simulink model "NLGC_1"  (R2017b)
settings: Solver=ode45  StartTime=0.0  StopTime=45  FixedStep=0.05  MaxStep=0.06  RelTol=1e-3  EnableMultiTasking=on
model workspace (MAT data in the model file):
  Sig = Simulink.Signal
  Sig.DataType = 'auto'
  Sig.Dimensions = -1
  Sig.DimensionsMode = 'auto'
  Sig.Complexity = 'auto'
  Sig.SampleTime = -1
  Sig.SamplingMode = 'auto'
undefined symbols (not defined in the file): IC, quadModel
libraries: simulink x4
Description:
  | This is a configurable quadcopter simulation.
  | This Simulink model demonstates position control.
  | 
  | Additional quadcopter modeling and simulation materials available at:
  | github.com/dch33/Quad-Sim
  | 
  | Copyright (C) 2014 D. Hartman, K. Landis, S. Moreno, J. Kim, M. Mehrer
  | 
  | License:
  |     This program is free software: you can redistribute it and/or modify
  |     it under the terms of the GNU LESSER GENERAL PUBLIC LICENSE as published by
  |     the Free Software Foundation, either version 3 of the License, or
  |     (at your option) any later version.
  | 
  |     This program is distributed in the hope that it will be useful,
  |     but WITHOUT ANY WARRANTY; without even the implied warranty of
  |     MERCHANTABILITY or FITNESS FOR A PARTICULAR PURPOSE.  See the
  |     GNU General Public License for more details.
  | 
  |     You should have received a copy of the GNU LESSER GENERAL PUBLIC LICENSE
  |     along with this program.  If not, see <http://www.gnu.org/licenses/>.
settings Model: ModifiedComment=hoang -- Wed Apr 11 06:13:36 2018 -- Version 1.7  Creator=David Hartman  LastModifiedBy=hoang
settings Model: ModifiedHistory=|
  | hoang -- Wed Apr 11 06:13:36 2018 -- Version 1.7
  | 
  | hoang -- Wed Apr 11 04:36:33 2018 -- Version 1.6
  | 
  | davidhartman -- Fri Jun 06 22:59:54 2014 -- Version 1.5
settings DataIOCC: SaveFormat=Array  SignalLogging=off
settings OptimizationCC: DefaultParameterBehavior=Inlined  LifeSpan=inf
settings DebuggingCC: SolverPrmCheckMsg=warning  UniqueDataStoreMsg=warning  StateNameClashWarn=warning  StrictBusMsg=ErrorOnBusTreatedAsVector  SFUnexpectedBacktrackingDiag=warning  SFNoUnconditionalDefaultTransitionDiag=warning  SFExecutionAtInitializationDiag=none
settings HardwareCC: ProdBitPerPointer=32  ProdBitPerSizeT=32  ProdBitPerPtrDiffT=32  ProdLargestAtomicFloat=None  ProdIntDivRoundTo=Undefined  ProdEndianess=Unspecified  ProdWordSize=32  ProdHWDeviceType=32-bit Generic
settings ModelReferenceCC: PropagateSignalLabelsOutOfModel=off
settings CodeAppCC: StateflowObjectComments=on
settings GRTTargetCC: TargetLangStandard=C89/C90 (ANSI)  GeneratePreprocessorConditionals=Disable all
settings ConfigComp: CovMetricSettings=dw  CovHtmlReporting=on  CovSaveCumulativeToWorkspaceVar=on  CovSaveSingleToWorkspaceVar=on  CovExternalEMLEnable=off

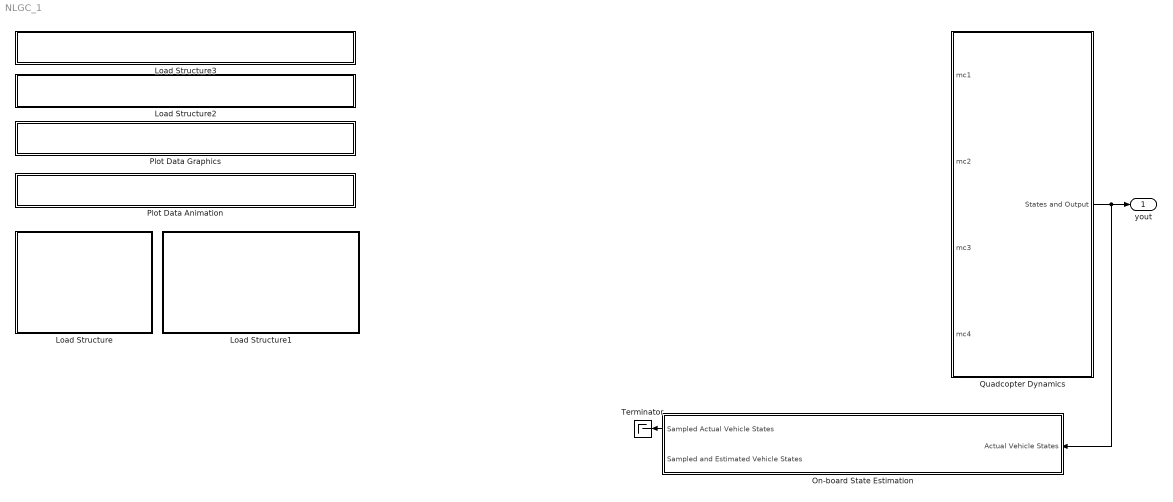
== system NLGC_1 ==
  Load Structure : Subsystem
      settings: OpenFcn=|
      | uiopen('load')
      | if ((exist('IC')==1) && (exist('quadModel')==1) && (exist('path')==1))
      | set_param(bdroot, 'SimulationCommand', 'update')
      | end
      mask Display: fprintf('LOAD:\nTimeseries\nPath\nCommands,\nQuadcopter\nModel, Or\nInitial\nConditions');
  Load Structure1 : Subsystem
      settings: OpenFcn=|
      | if (exist('IC')==1 && exist('quadModel')==1 && exist('yout') && exist('tout'))
      | saveSimResults()
      | else
      | msgbox('No Data To Save!')
      | end
      mask Display: fprintf('SAVE:\nSimulation\nResults');
  Load Structure2 : Subsystem
      settings: OpenFcn=|
      | if exist('GUI_Modeling') == 2,
      | run('GUI_Modeling')
      | 
      | else
      | 
      | msgbox('The desired GUI must be first added to MATLABs path.')
      | 
      | end
      mask Display: fprintf('OPEN GUI: Build New \n Model');
  Load Structure3 : Subsystem
      settings: OpenFcn=|
      | if exist('GUI_IC') == 2,
      | run('GUI_IC')
      | 
      | else
      | 
      | msgbox('The desired GUI must be first added to MATLABs path.')
      | 
      | end
      mask Display: fprintf('OPEN GUI: Create Initial \n Conditions');
  On-board State Estimation : Subsystem  mask{ControllerSampleTime=1/350, Gyro_Alpha=0.50, Accel_Alpha=0.06, EAComp=0.92}
      mask prompts: ControllerSampleTime "State sensor sampling time (s):"; Gyro_Alpha "Gyro Alpha Value:"; Accel_Alpha "Accelerometer Alpha Value:"; EAComp "Complimentary Filter Alpha (must be between 0 and 1):"
      mask Help:
      | Sampling Time: A typical value might be 0.02 to 0.002 seconds (50 Hz to 400 Hz)
      | depending on the control system and sensors used. For best simulink performance,
      | it may be necessarry to round the value a bit to achieve an integer multiple
      | relationship between motor command sampling time and state estimation sampling time.
      | See simulink documentation for more details.
      mask TypeOptions ControllerSampleTime: Rate Transition/OutPortSampleTime
      mask TypeOptions Gyro_Alpha: filterRawData()/Gyro_Alpha
      mask TypeOptions Accel_Alpha: filterRawData()/Accel_Alpha
      mask TypeOptions EAComp: State Estimation and Complimentary Mixing/EAComp
      mask Display:
      | fprintf(['Sampling Time: ' num2str(ControllerSampleTime) ' (s)']);
      | fprintf(['\n \n' num2str(1/ControllerSampleTime) ' Hz']);
  Plot Data Animation : Subsystem
      settings: OpenFcn=|
      | if exist('QuadAnim4') == 2,
      |     if exist('yout')
      | 	run('QuadAnim4');
      |     else
      |     msgbox('Simulation must be run before data can be plotted.');
      |     end
      | else                                                                          msgbox('The desired GUI must be first added to MATLABs path.')
      | end
      mask Display: fprintf('OPEN GUI: Flight Animation')
  Plot Data Graphics : Subsystem
      settings: OpenFcn=|
      | if exist('yout')
      | yout = evalin('base', 'yout');
      | tout = evalin('base', 'tout');
      | quadPlots(yout, tout)
      | else
      | msgbox('Simulation must be run before data can be plotted.')
      | end
      mask Display: fprintf('OPEN PLOT: State Data')
  Quadcopter Dynamics : Subsystem
  Terminator : Terminator
  yout : Outport
  wires:
  Quadcopter Dynamics/1(States and Output) -> yout/1, On-board State Estimation/1(Actual Vehicle States)
  On-board State Estimation/1(Sampled Actual Vehicle States) -> Terminator/1

== system NLGC_1/Load Structure ==

== system NLGC_1/Load Structure1 ==

== system NLGC_1/Load Structure2 ==

== system NLGC_1/Load Structure3 ==

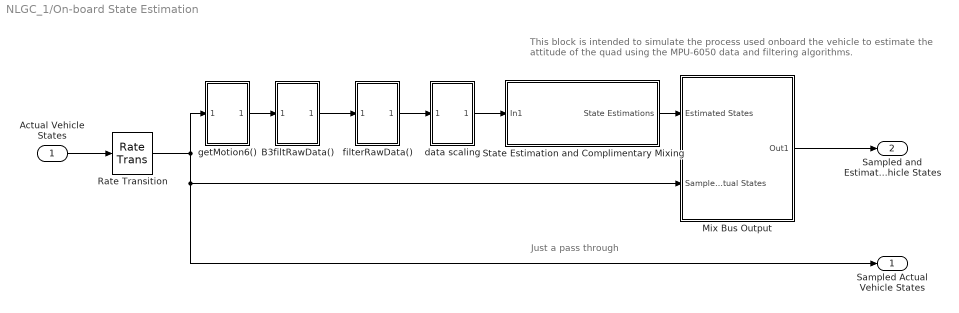
== system NLGC_1/On-board State Estimation ==
  note: This block is intended to simulate the process used onboard the vehicle
      | to estimate the attitude of the quad using the MPU-6050 data and filtering algorithms.
  note: Just a pass through
  Actual Vehicle States : Inport
  B3filtRawData() : Subsystem  mask{inputGain=1/3.102185882e+03, x1x2Gain=3, y2Gain=2.7130114176, y1Gain=-2.4657422174, y0Gain=0.7501519731}
      mask prompts: inputGain "Input Gain:"; x1x2Gain "x1x2 Gain:"; y2Gain "y2 Gain:"; y1Gain "y1 Gain:"; y0Gain "y0 Gain:"
      mask TypeOptions inputGain: InputGain/Gain
      mask TypeOptions x1x2Gain: x1x2Gain/Gain
      mask TypeOptions y2Gain: y2Gain/Gain
      mask TypeOptions y1Gain: y1Gain/Gain
      mask TypeOptions y0Gain: y0Gain/Gain
  Mix Bus Output : Subsystem
  Rate Transition : RateTransition  Deterministic=off  OutPortSampleTime=ControllerSampleTime
  State Estimation and Complimentary Mixing : Subsystem  mask{EAComp=EAComp}
      mask prompts: EAComp "Complimentary Filter Alpha:"
      mask TypeOptions EAComp: Complimentary Filter/EAComp
  data scaling : Subsystem
  filterRawData() : Subsystem  mask{Gyro_Alpha=Gyro_Alpha, Accel_Alpha=Accel_Alpha}
      mask prompts: Gyro_Alpha "Gyro Alpha Value:"; Accel_Alpha "Accelerometer Alpha Value:"
      mask TypeOptions Gyro_Alpha: Gyro alpha/Gain
      mask TypeOptions Accel_Alpha: Accel alpha/Gain
  getMotion6() : Subsystem
  Sampled Actual Vehicle States : Outport
  Sampled and Estimated Vehicle States : Outport  Port=2
  wires:
  Actual Vehicle States/1 -> Rate Transition/1
  Rate Transition/1 -> getMotion6()/1(In1), Sampled Actual Vehicle States/1, Mix Bus Output/2(Sampled Actual States)
  getMotion6()/1(Out1) -> B3filtRawData()/1(In1)
  data scaling/1(Out1) -> State Estimation and Complimentary Mixing/1(In1)
  State Estimation and Complimentary Mixing/1(State Estimations) -> Mix Bus Output/1(Estimated States)
  Mix Bus Output/1(Out1) -> Sampled and Estimated Vehicle States/1
  B3filtRawData()/1(Out1) -> filterRawData()/1(In1)
  filterRawData()/1(Out1) -> data scaling/1(In1)

== system NLGC_1/Plot Data Animation ==

== system NLGC_1/Plot Data Graphics ==

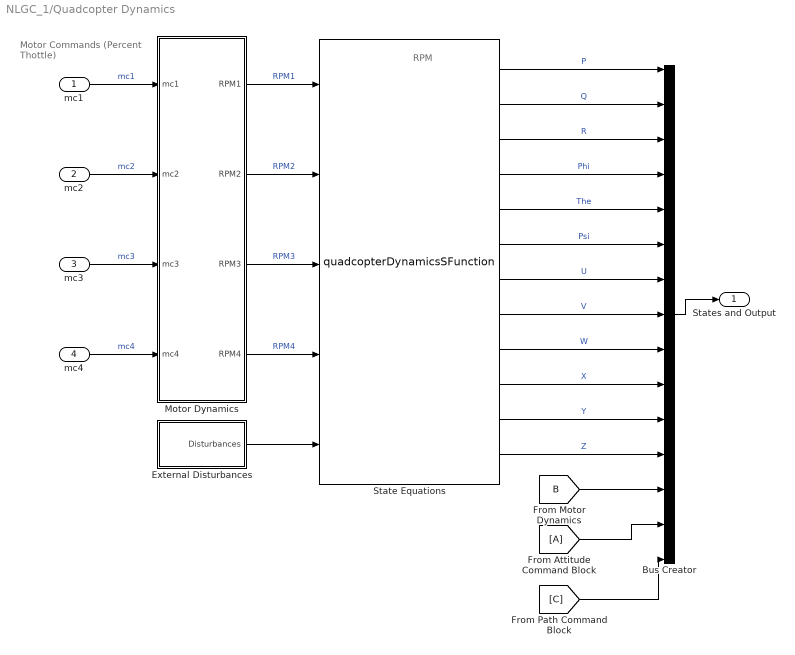
== system NLGC_1/Quadcopter Dynamics ==
  note: RPM
  note: Motor Commands
      | (Percent Thottle)
  mc1 : Inport
  mc2 : Inport  Port=2
  mc3 : Inport  Port=3
  mc4 : Inport  Port=4
  Bus Creator : BusCreator  Inputs='P','Q','R','Phi','The','Psi','U','V','W','X','Y','Z','mc and RPM','Attitude_Cmd','XY_Cmd'
  External Disturbances : Subsystem
  Motor Dynamics : Subsystem
  State Equations : M-S-Function  FunctionName=quadcopterDynamicsSFunction  Parameters=quadModel, IC
      mask Display:
      | port_label('input', 1, 'RPM1')
      | port_label('input', 2, 'RPM2')
      | port_label('input', 3, 'RPM3')
      | port_label('input', 4, 'RPM4')
      | port_label('input', 5, 'Disturbances')
      | port_label('output', 1, 'P')
      | port_label('output', 2, 'Q')
      | port_label('output', 3, 'R')
      | port_label('output', 4, 'Phi')
      | port_label('output', 5, 'The')
      | port_label('output', 6, 'Psi')
      | port_label('output', 7, 'U')
      | port_label('output', 8, 'V')
      | port_label('output', 9, 'W')
      | port_label('output', 10, 'X')
      | port_label('output', 11, 'Y')
      | port_label('output', 12, 'Z')
  States and Output : Outport
  wires:
  State Equations/1 -> Bus Creator/1  "P"
  State Equations/2 -> Bus Creator/2  "Q"
  State Equations/3 -> Bus Creator/3  "R"
  State Equations/4 -> Bus Creator/4  "Phi"
  State Equations/5 -> Bus Creator/5  "The"
  State Equations/6 -> Bus Creator/6  "Psi"
  State Equations/7 -> Bus Creator/7  "U"
  State Equations/8 -> Bus Creator/8  "V"
  State Equations/9 -> Bus Creator/9  "W"
  State Equations/10 -> Bus Creator/10  "X"
  State Equations/11 -> Bus Creator/11  "Y"
  State Equations/12 -> Bus Creator/12  "Z"
  Bus Creator/1 -> States and Output/1
  Motor Dynamics/1(RPM1) -> State Equations/1  "RPM1"
  Motor Dynamics/2(RPM2) -> State Equations/2  "RPM2"
  Motor Dynamics/3(RPM3) -> State Equations/3  "RPM3"
  Motor Dynamics/4(RPM4) -> State Equations/4  "RPM4"
  mc1/1 -> Motor Dynamics/1(mc1)  "mc1"
  mc4/1 -> Motor Dynamics/4(mc4)  "mc4"
  mc3/1 -> Motor Dynamics/3(mc3)  "mc3"
  mc2/1 -> Motor Dynamics/2(mc2)  "mc2"
  External Disturbances/1("Disturbances ") -> State Equations/5
  [A] -> Bus Creator/14
  [B] -> Bus Creator/13
  [C] -> Bus Creator/15

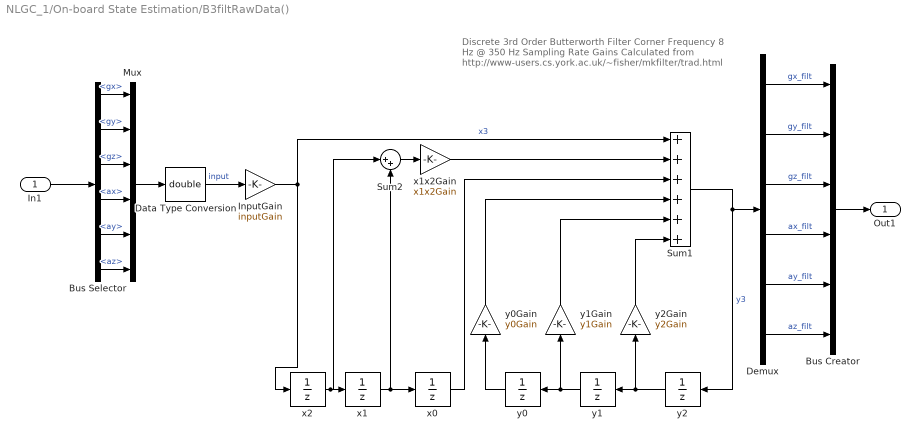
== system NLGC_1/On-board State Estimation/B3filtRawData() ==
  note: Discrete
      | 3rd Order Butterworth Filter
      | Corner Frequency 8 Hz @ 350 Hz Sampling Rate
      | Gains Calculated from
      | http://www-users.cs.york.ac.uk/~fisher/mkfilter/trad.html
  In1 : Inport
  Bus Creator : BusCreator  Inputs=6
  Bus Selector : BusSelector  OutputSignals=gx,gy,gz,ax,ay,az
  Data Type Conversion : DataTypeConversion  OutDataTypeStr=double  RndMeth=Nearest
  Demux : Demux  Outputs=6
  InputGain : Gain  Gain=inputGain
  Mux : Mux  Inputs=6
  Sum1 : Sum  Inputs=++++++
  Sum2 : Sum  Inputs=|++
  x0 : UnitDelay  SampleTime=-1
  x1 : UnitDelay  SampleTime=-1
  x1x2Gain : Gain  Gain=x1x2Gain
  x2 : UnitDelay  SampleTime=-1
  y0 : UnitDelay  SampleTime=-1
  y0Gain : Gain  Gain=y0Gain
  y1 : UnitDelay  SampleTime=-1
  y1Gain : Gain  Gain=y1Gain
  y2 : UnitDelay  SampleTime=-1
  y2Gain : Gain  Gain=y2Gain
  Out1 : Outport
  wires:
  Sum1/1 -> Demux/1, y2/1  "y3"
  In1/1 -> Bus Selector/1
  Bus Selector/1 -> Mux/1  "<gx>"
  Bus Selector/2 -> Mux/2  "<gy>"
  Bus Selector/3 -> Mux/3  "<gz>"
  Mux/1 -> Data Type Conversion/1
  Demux/1 -> Bus Creator/1  "gx_filt"
  Demux/2 -> Bus Creator/2  "gy_filt"
  Demux/3 -> Bus Creator/3  "gz_filt"
  Bus Creator/1 -> Out1/1
  Data Type Conversion/1 -> InputGain/1  "input"
  Bus Selector/4 -> Mux/4  "<ax>"
  Bus Selector/5 -> Mux/5  "<ay>"
  Bus Selector/6 -> Mux/6  "<az>"
  Demux/4 -> Bus Creator/4  "ax_filt"
  Demux/5 -> Bus Creator/5  "ay_filt"
  Demux/6 -> Bus Creator/6  "az_filt"
  y2/1 -> y2Gain/1, y1/1
  y1/1 -> y1Gain/1, y0/1
  InputGain/1 -> x2/1, Sum1/1  "x3"
  x2/1 -> Sum2/1, x1/1
  x1/1 -> Sum2/2, x0/1
  Sum2/1 -> x1x2Gain/1
  x1x2Gain/1 -> Sum1/2
  y0Gain/1 -> Sum1/4
  y0/1 -> y0Gain/1
  y1Gain/1 -> Sum1/5
  y2Gain/1 -> Sum1/6
  x0/1 -> Sum1/3

== system NLGC_1/On-board State Estimation/Mix Bus Output ==
  note: These states are sampled actual values
      | not used by the stability controller
  note: These are the estimated states
  Estimated States : Inport
  Sampled Actual States : Inport  Port=2
  Bus Creator : BusCreator  Inputs=12
  Bus Selector1 : BusSelector  OutputSignals=U,V,W,X,Y,Z
  Bus Selector2 : BusSelector  OutputSignals=P,Q,R,Phi,The,Psi
  Debug Scopes For Comparing Actual Versus Estimated Outputs This illustrates some of the effects from filtering : Subsystem
  Out1 : Outport
  wires:
  Bus Selector2/2 -> Bus Creator/2  "<Q>"
  Bus Selector2/3 -> Bus Creator/3  "<R>"
  Bus Selector2/1 -> Bus Creator/1  "<P>"
  Bus Selector2/5 -> Bus Creator/5  "<The>"
  Bus Selector1/5 -> Bus Creator/11  "<Y>"
  Bus Selector1/4 -> Bus Creator/10  "<X>"
  Bus Selector1/1 -> Bus Creator/7  "<U>"
  Estimated States/1 -> Debug Scopes For Comparing Actual Versus Estimated Outputs This illustrates some of the effects from filtering/1(Estimated), Bus Selector2/1
  Bus Selector2/4 -> Bus Creator/4  "<Phi>"
  Bus Selector1/2 -> Bus Creator/8  "<V>"
  Bus Selector1/6 -> Bus Creator/12  "<Z>"
  Bus Creator/1 -> Out1/1
  Sampled Actual States/1 -> Debug Scopes For Comparing Actual Versus Estimated Outputs This illustrates some of the effects from filtering/2(Actual), Bus Selector1/1
  Bus Selector1/3 -> Bus Creator/9  "<W>"
  Bus Selector2/6 -> Bus Creator/6  "<Psi>"

== system NLGC_1/On-board State Estimation/State Estimation and Complimentary Mixing ==
  note: The specific state estimation procedure employed in these bocks is
      | to be considered experimental (like everything else in this simulation).
      | While functional within the context of our application, this is not to be taken
      | as a "correct" method for state estimation or gyro/accelerometer data combination.
  note: Note:
      | x_gyro is taken as P,
      | y_gyro as Q,
      | z_gyro ad R.
  In1 : Inport
  Bus Creator : BusCreator  Inputs=6
  Bus Selector : BusSelector  OutputSignals=P,Q,R,x_acc,y_acc,z_acc
  Complimentary Filter : Subsystem  mask{EAComp=EAComp}
      mask prompts: EAComp "Complimentary Filter Alpha:"
      mask TypeOptions EAComp: EAComp1/Gain
  Subsystem : Subsystem
  Subsystem1 : Subsystem
  State Estimations : Outport
  wires:
  In1/1 -> Bus Selector/1
  Bus Selector/1 -> Bus Creator/4, Subsystem/3(P)  "<P>"
  Bus Selector/3 -> Bus Creator/6, Subsystem/5(R)  "<R>"
  Bus Selector/2 -> Bus Creator/5, Subsystem/4(Q)  "<Q>"
  Subsystem/2(thetaDot_gyro) -> Complimentary Filter/2(theDot_gyro)  "thateDot_gyro"
  Subsystem/3(psiDot_gyro) -> Complimentary Filter/3(psiDot_gyro)  "psiDot_gyro"
  Subsystem/1(phiDot_gyro) -> Complimentary Filter/1(phiDot_gyro)  "phiDot_gyro"
  Complimentary Filter/1(phi_est) -> Bus Creator/1, Subsystem/1(Phi)  "Phi"
  Complimentary Filter/2(theta_est) -> Bus Creator/2, Subsystem/2(Theta)  "The"
  Complimentary Filter/3(psi_est) -> Bus Creator/3  "Psi"
  Subsystem1/2(phi_acc) -> Complimentary Filter/5(phiDot_acc)  "phi_acc"
  Subsystem1/1(theta_acc) -> Complimentary Filter/4(the_acc)  "theta_acc"
  Bus Selector/4 -> Subsystem1/1(x_acc)  "<x_acc>"
  Bus Selector/5 -> Subsystem1/2(y_acc)  "<y_acc>"
  Bus Selector/6 -> Subsystem1/3(z_acc)  "<z_acc>"
  Bus Creator/1 -> State Estimations/1

== system NLGC_1/On-board State Estimation/data scaling ==
  note: For simulation, no
      | offset value is calculated.
  In1 : Inport
  Bus Creator : BusCreator  Inputs=6
  Bus Selector : BusSelector  OutputSignals=gx_filt,gy_filt,gz_filt,ax_filt,ay_filt,az_filt
  Demux : Demux  Outputs=3
  Demux1 : Demux  Outputs=3
  Gain : Gain  Gain=pi/(180*131)
  Gain1 : Gain  Gain=9.81*16384
  Mux1 : Mux  Inputs=3
  Mux2 : Mux  Inputs=3
  Out1 : Outport
  wires:
  In1/1 -> Bus Selector/1
  Bus Selector/1 -> Mux1/1  "<gx_filt>"
  Bus Selector/2 -> Mux1/2  "<gy_filt>"
  Bus Selector/3 -> Mux1/3  "<gz_filt>"
  Bus Selector/4 -> Mux2/1  "<ax_filt>"
  Bus Selector/5 -> Mux2/2  "<ay_filt>"
  Bus Selector/6 -> Mux2/3  "<az_filt>"
  Mux2/1 -> Gain1/1
  Mux1/1 -> Gain/1
  Gain1/1 -> Demux1/1
  Gain/1 -> Demux/1
  Demux/1 -> Bus Creator/1  "P"
  Demux/2 -> Bus Creator/2  "Q"
  Demux/3 -> Bus Creator/3  "R"
  Demux1/1 -> Bus Creator/4  "x_acc"
  Demux1/2 -> Bus Creator/5  "y_acc"
  Demux1/3 -> Bus Creator/6  "z_acc"
  Bus Creator/1 -> Out1/1

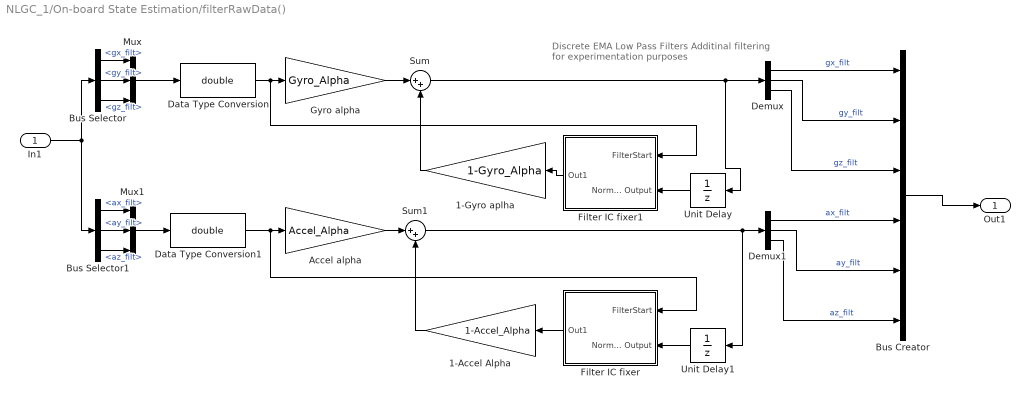
== system NLGC_1/On-board State Estimation/filterRawData() ==
  note: Discrete EMA
      | Low Pass Filters
      | Additinal filtering for experimentation purposes
  In1 : Inport
  1-Accel Alpha : Gain  Gain=1-Accel_Alpha
  1-Gyro aplha : Gain  Gain=1-Gyro_Alpha
  Accel alpha : Gain  Gain=Accel_Alpha
  Bus Creator : BusCreator  Inputs=6
  Bus Selector : BusSelector  OutputSignals=gx_filt,gy_filt,gz_filt
  Bus Selector1 : BusSelector  OutputSignals=ax_filt,ay_filt,az_filt
  Data Type Conversion : DataTypeConversion  OutDataTypeStr=double  RndMeth=Nearest
  Data Type Conversion1 : DataTypeConversion  OutDataTypeStr=double  RndMeth=Nearest
  Demux : Demux  Outputs=3
  Demux1 : Demux  Outputs=3
  Filter IC fixer : Subsystem
  Filter IC fixer1 : Subsystem
  Gyro alpha : Gain  Gain=Gyro_Alpha
  Mux : Mux  Inputs=3
  Mux1 : Mux  Inputs=3
  Sum : Sum  Inputs=|++
  Sum1 : Sum  Inputs=|++
  Unit Delay : UnitDelay  SampleTime=-1
  Unit Delay1 : UnitDelay  SampleTime=-1
  Out1 : Outport
  wires:
  Gyro alpha/1 -> Sum/1
  Sum/1 -> Demux/1, Unit Delay/1
  In1/1 -> Bus Selector1/1, Bus Selector/1
  Accel alpha/1 -> Sum1/1
  1-Gyro aplha/1 -> Sum/2
  1-Accel Alpha/1 -> Sum1/2
  Unit Delay1/1 -> Filter IC fixer/2(Normal Output)
  Filter IC fixer/1(Out1) -> 1-Accel Alpha/1
  Unit Delay/1 -> Filter IC fixer1/2(Normal Output)
  Filter IC fixer1/1(Out1) -> 1-Gyro aplha/1
  Bus Selector/1 -> Mux/1  "<gx_filt>"
  Bus Selector/2 -> Mux/2  "<gy_filt>"
  Bus Selector/3 -> Mux/3  "<gz_filt>"
  Mux/1 -> Data Type Conversion/1
  Demux/1 -> Bus Creator/1  "gx_filt"
  Demux/2 -> Bus Creator/2  "gy_filt"
  Demux/3 -> Bus Creator/3  "gz_filt"
  Bus Creator/1 -> Out1/1
  Mux1/1 -> Data Type Conversion1/1
  Bus Selector1/1 -> Mux1/1  "<ax_filt>"
  Bus Selector1/2 -> Mux1/2  "<ay_filt>"
  Bus Selector1/3 -> Mux1/3  "<az_filt>"
  Sum1/1 -> Unit Delay1/1, Demux1/1
  Demux1/1 -> Bus Creator/4  "ax_filt"
  Demux1/2 -> Bus Creator/5  "ay_filt"
  Demux1/3 -> Bus Creator/6  "az_filt"
  Data Type Conversion/1 -> Filter IC fixer1/1(FilterStart), Gyro alpha/1
  Data Type Conversion1/1 -> Filter IC fixer/1(FilterStart), Accel alpha/1

== system NLGC_1/On-board State Estimation/getMotion6() ==
  note: Simulate getMotion()
  note: Get std measurement from sensor
      | connect to front mask
  In1 : Inport
  Accelerometer : Subsystem
  Bus Creator : BusCreator  Inputs=6
  Bus Selector : BusSelector  OutputSignals=P,Q,R,Phi,The
  Gyro signals : Subsystem
  Out1 : Outport
  wires:
  Bus Selector/2 -> Gyro signals/2(Q)  "<Q>"
  Bus Selector/1 -> Gyro signals/1(P)  "<P>"
  Gyro signals/2(gy) -> Bus Creator/2  "gy"
  Accelerometer/1(ax) -> Bus Creator/4  "ax"
  Bus Selector/5 -> Accelerometer/2(Theta)  "<The>"
  Bus Selector/4 -> Accelerometer/1(Phi)  "<Phi>"
  Bus Selector/3 -> Gyro signals/3(R)  "<R>"
  Gyro signals/1(gx) -> Bus Creator/1  "gx"
  In1/1 -> Bus Selector/1
  Gyro signals/3(gz) -> Bus Creator/3  "gz"
  Accelerometer/2(ay) -> Bus Creator/5  "ay"
  Accelerometer/3(az) -> Bus Creator/6  "az"
  Bus Creator/1 -> Out1/1

== system NLGC_1/Quadcopter Dynamics/External Disturbances ==
  note: Note: Torques are in units of N*m, Forces in N
      | Torques are applied to the BODY coordinate system.
      | Forces are applied from the WORLD coordinate system!
      | This can be changed by adjusting the equations within the S-function.
  Bus Creator : BusCreator  Inputs=6
  Bus to Vector : BusToVector
  Constant{2..6} (5 alike) : Constant  Value=0
  Step : Step  After=0  SampleTime=0
  "Disturbances " : Outport
  wires:
  Bus to Vector/1 -> "Disturbances "/1
  Bus Creator/1 -> Bus to Vector/1
  Constant6/1 -> Bus Creator/1  "Tau_bx-axis"
  Step/1 -> Bus Creator/2  "Tau_by-axis"
  Constant2/1 -> Bus Creator/3  "Tau_bz-axis"
  Constant3/1 -> Bus Creator/4  "Force_x-axis"
  Constant4/1 -> Bus Creator/5  "Force_y-axis"
  Constant5/1 -> Bus Creator/6  "Force_z-axis"

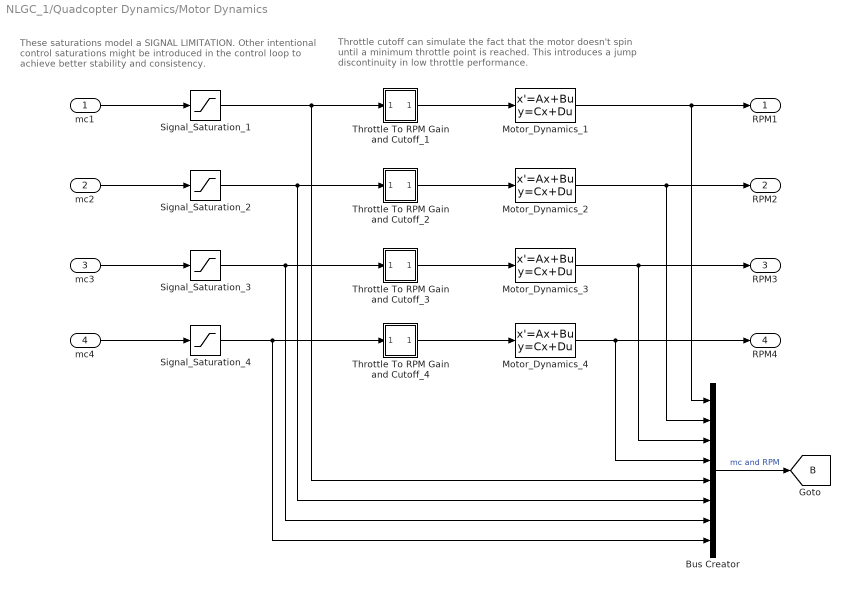
== system NLGC_1/Quadcopter Dynamics/Motor Dynamics ==
  note: Throttle cutoff can simulate the fact that the motor doesn't
      | spin until a minimum throttle point is reached. This introduces
      | a jump discontinuity in low throttle performance.
  note: These saturations model a SIGNAL LIMITATION.
      | Other intentional control saturations might be introduced in the
      | control loop to achieve better stability and consistency.
  mc1 : Inport
  mc2 : Inport  Port=2
  mc3 : Inport  Port=3
  mc4 : Inport  Port=4
  Bus Creator : BusCreator  Inputs=8
  Motor_Dynamics_1 : StateSpace  A=-1/quadModel.T  C=1/quadModel.T  D=0  InitialCondition=IC.w1*quadModel.T
  Motor_Dynamics_2 : StateSpace  A=-1/quadModel.T  C=1/quadModel.T  D=0  InitialCondition=IC.w2*quadModel.T
  Motor_Dynamics_3 : StateSpace  A=-1/quadModel.T  C=1/quadModel.T  D=0  InitialCondition=IC.w3*quadModel.T
  Motor_Dynamics_4 : StateSpace  A=-1/quadModel.T  C=1/quadModel.T  D=0  InitialCondition=IC.w4*quadModel.T
  Signal_Saturation_{1..4} (4 alike) : Saturate  UpperLimit=100  LowerLimit=0
  Throttle To RPM Gain and Cutoff_1 : Subsystem
  Throttle To RPM Gain and Cutoff_2 : Subsystem
  Throttle To RPM Gain and Cutoff_3 : Subsystem
  Throttle To RPM Gain and Cutoff_4 : Subsystem
  RPM1 : Outport
  RPM2 : Outport  Port=2
  RPM3 : Outport  Port=3
  RPM4 : Outport  Port=4
  tag scope: B=global
  wires:
  mc1/1 -> Signal_Saturation_1/1
  mc4/1 -> Signal_Saturation_4/1
  mc2/1 -> Signal_Saturation_2/1
  mc3/1 -> Signal_Saturation_3/1
  Signal_Saturation_1/1 -> Bus Creator/5, Throttle To RPM Gain and Cutoff_1/1(In5)
  Signal_Saturation_2/1 -> Bus Creator/6, Throttle To RPM Gain and Cutoff_2/1(In5)
  Signal_Saturation_3/1 -> Bus Creator/7, Throttle To RPM Gain and Cutoff_3/1(In5)
  Signal_Saturation_4/1 -> Bus Creator/8, Throttle To RPM Gain and Cutoff_4/1(In5)
  Throttle To RPM Gain and Cutoff_1/1(Out5) -> Motor_Dynamics_1/1
  Throttle To RPM Gain and Cutoff_2/1(Out5) -> Motor_Dynamics_2/1
  Throttle To RPM Gain and Cutoff_3/1(Out5) -> Motor_Dynamics_3/1
  Throttle To RPM Gain and Cutoff_4/1(Out5) -> Motor_Dynamics_4/1
  Motor_Dynamics_1/1 -> Bus Creator/1, RPM1/1
  Motor_Dynamics_2/1 -> Bus Creator/2, RPM2/1
  Motor_Dynamics_3/1 -> Bus Creator/3, RPM3/1
  Motor_Dynamics_4/1 -> Bus Creator/4, RPM4/1
  Bus Creator/1 -> [B]  "mc and RPM"

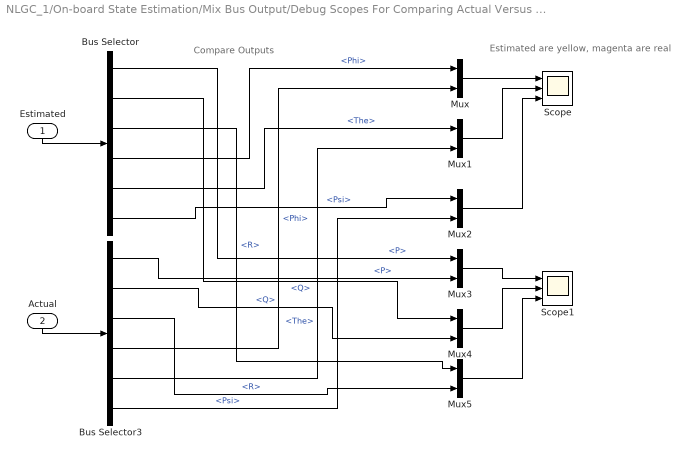
== system NLGC_1/On-board State Estimation/Mix Bus Output/Debug Scopes For Comparing Actual Versus Estimated Outputs This illustrates some of the effects from filtering ==
  note: Estimated are yellow, magenta are real
  note: Compare Outputs
  Estimated : Inport
  Actual : Inport  Port=2
  Bus Selector : BusSelector  OutputSignals=P,Q,R,Phi,The,Psi
  Bus Selector3 : BusSelector  OutputSignals=P,Q,R,Phi,The,Psi
  Mux{,1..5} (6 alike) : Mux  Inputs=2
  Scope : Scope  NumInputPorts=3
  Scope1 : Scope  NumInputPorts=3
  wires:
  Actual/1 -> Bus Selector3/1
  Mux5/1 -> Scope1/3
  Estimated/1 -> Bus Selector/1
  Bus Selector3/2 -> Mux4/2  "<Q>"
  Mux3/1 -> Scope1/1
  Mux4/1 -> Scope1/2
  Bus Selector/1 -> Mux3/1  "<P>"
  Bus Selector3/1 -> Mux3/2  "<P>"
  Bus Selector3/5 -> Mux1/2  "<The>"
  Bus Selector/3 -> Mux5/1  "<R>"
  Bus Selector/6 -> Mux2/1  "<Psi>"
  Bus Selector/2 -> Mux4/1  "<Q>"
  Mux2/1 -> Scope/3
  Bus Selector/5 -> Mux1/1  "<The>"
  Bus Selector/4 -> Mux/1  "<Phi>"
  Bus Selector3/3 -> Mux5/2  "<R>"
  Bus Selector3/6 -> Mux2/2  "<Psi>"
  Mux/1 -> Scope/1
  Mux1/1 -> Scope/2
  Bus Selector3/4 -> Mux/2  "<Phi>"

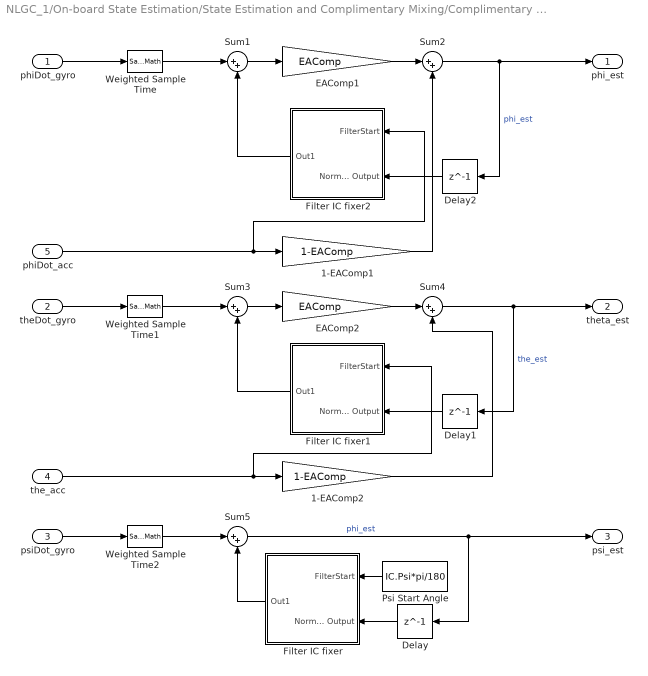
== system NLGC_1/On-board State Estimation/State Estimation and Complimentary Mixing/Complimentary Filter ==
  phiDot_gyro : Inport
  theDot_gyro : Inport  Port=2
  psiDot_gyro : Inport  Port=3
  the_acc : Inport  Port=4
  phiDot_acc : Inport  Port=5
  1-EAComp1 : Gain  Gain=1-EAComp
  1-EAComp2 : Gain  Gain=1-EAComp
  Delay : Delay  DelayLength=1  InitialCondition=0
  Delay1 : Delay  DelayLength=1  InitialCondition=0
  Delay2 : Delay  DelayLength=1  InitialCondition=0
  EAComp1 : Gain  Gain=EAComp
  EAComp2 : Gain  Gain=EAComp
  Filter IC fixer : Subsystem
  Filter IC fixer1 : Subsystem
  Filter IC fixer2 : Subsystem
  Psi Start Angle : Constant  Value=IC.Psi*pi/180
  Sum{1..5} (5 alike) : Sum  Inputs=|++
  Weighted Sample Time : SampleTimeMath  TsampMathOp=*
  Weighted Sample Time1 : SampleTimeMath  TsampMathOp=*
  Weighted Sample Time2 : SampleTimeMath  TsampMathOp=*
  phi_est : Outport
  theta_est : Outport  Port=2
  psi_est : Outport  Port=3
  wires:
  Weighted Sample Time/1 -> Sum1/1
  Sum1/1 -> EAComp1/1
  Sum2/1 -> Delay2/1, phi_est/1  "phi_est"
  1-EAComp1/1 -> Sum2/2
  phiDot_gyro/1 -> Weighted Sample Time/1
  phiDot_acc/1 -> Filter IC fixer2/1(FilterStart), 1-EAComp1/1
  EAComp1/1 -> Sum2/1
  Weighted Sample Time1/1 -> Sum3/1
  Sum3/1 -> EAComp2/1
  Sum4/1 -> Delay1/1, theta_est/1  "the_est"
  1-EAComp2/1 -> Sum4/2
  theDot_gyro/1 -> Weighted Sample Time1/1
  the_acc/1 -> 1-EAComp2/1, Filter IC fixer1/1(FilterStart)
  EAComp2/1 -> Sum4/1
  psiDot_gyro/1 -> Weighted Sample Time2/1
  Weighted Sample Time2/1 -> Sum5/1
  Sum5/1 -> Delay/1, psi_est/1  "phi_est"
  Delay/1 -> Filter IC fixer/2(Normal Output)
  Filter IC fixer/1(Out1) -> Sum5/2
  Psi Start Angle/1 -> Filter IC fixer/1(FilterStart)
  Filter IC fixer1/1(Out1) -> Sum3/2
  Filter IC fixer2/1(Out1) -> Sum1/2
  Delay1/1 -> Filter IC fixer1/2(Normal Output)
  Delay2/1 -> Filter IC fixer2/2(Normal Output)

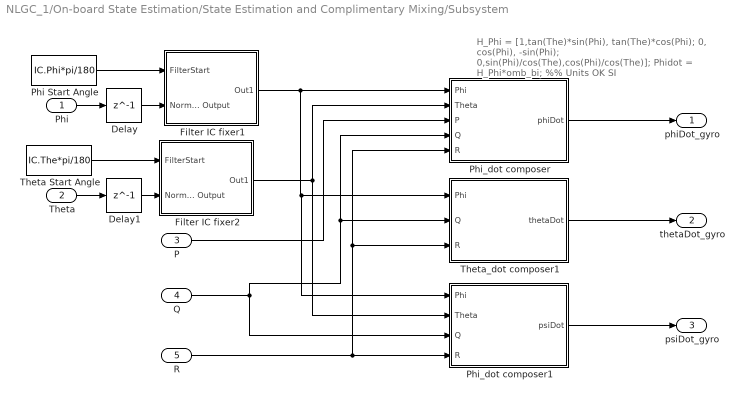
== system NLGC_1/On-board State Estimation/State Estimation and Complimentary Mixing/Subsystem ==
  note: H_Phi = [1,tan(The)*sin(Phi), tan(The)*cos(Phi);
      |          0,         cos(Phi),         -sin(Phi);
      |          0,sin(Phi)/cos(The),cos(Phi)/cos(The)];
      | Phidot = H_Phi*omb_bi; %% Units OK SI
  Phi : Inport
  Theta : Inport  Port=2
  P : Inport  Port=3
  Q : Inport  Port=4
  R : Inport  Port=5
  Delay : Delay  DelayLength=1  InitialCondition=0
  Delay1 : Delay  DelayLength=1  InitialCondition=0
  Filter IC fixer1 : Subsystem
  Filter IC fixer2 : Subsystem
  Phi Start Angle : Constant  Value=IC.Phi*pi/180
  Phi_dot composer : Subsystem
  Phi_dot composer1 : Subsystem
  Theta Start Angle : Constant  Value=IC.The*pi/180
  Theta_dot composer1 : Subsystem
  phiDot_gyro : Outport
  thetaDot_gyro : Outport  Port=2
  psiDot_gyro : Outport  Port=3
  wires:
  P/1 -> Phi_dot composer/3(P)
  Q/1 -> Phi_dot composer1/3(Q), Theta_dot composer1/2(Q), Phi_dot composer/4(Q)
  Phi_dot composer/1(phiDot) -> phiDot_gyro/1
  Theta_dot composer1/1(thetaDot) -> thetaDot_gyro/1
  R/1 -> Theta_dot composer1/3(R), Phi_dot composer/5(R), Phi_dot composer1/4(R)
  Phi_dot composer1/1(psiDot) -> psiDot_gyro/1
  Filter IC fixer1/1(Out1) -> Phi_dot composer1/1(Phi), Theta_dot composer1/1(Phi), Phi_dot composer/1(Phi)
  Delay/1 -> Filter IC fixer1/2(Normal Output)
  Phi/1 -> Delay/1
  Phi Start Angle/1 -> Filter IC fixer1/1(FilterStart)
  Theta/1 -> Delay1/1
  Filter IC fixer2/1(Out1) -> Phi_dot composer/2(Theta), Phi_dot composer1/2(Theta)
  Delay1/1 -> Filter IC fixer2/2(Normal Output)
  Theta Start Angle/1 -> Filter IC fixer2/1(FilterStart)

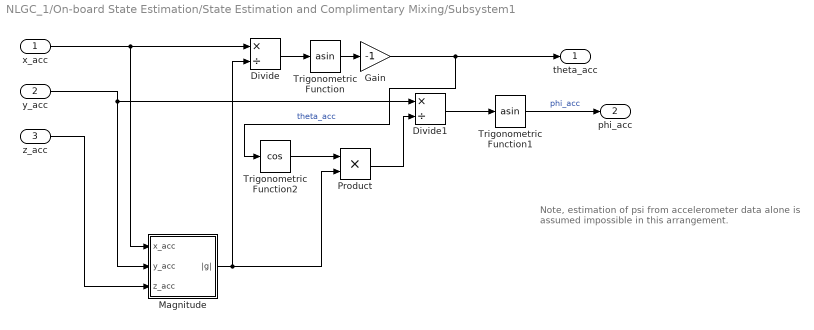
== system NLGC_1/On-board State Estimation/State Estimation and Complimentary Mixing/Subsystem1 ==
  note: Note, estimation of psi from accelerometer data alone
      | is assumed impossible in this arrangement.
  x_acc : Inport
  y_acc : Inport  Port=2
  z_acc : Inport  Port=3
  Divide : Product  Inputs=*/
  Divide1 : Product  Inputs=*/
  Gain : Gain  Gain=-1
  Magnitude : Subsystem
  Product : Product
  Trigonometric Function : Trigonometry  Operator=asin  OutputSignalType=real
  Trigonometric Function1 : Trigonometry  Operator=asin  OutputSignalType=real
  Trigonometric Function2 : Trigonometry  Operator=cos  OutputSignalType=real
  theta_acc : Outport
  phi_acc : Outport  Port=2
  wires:
  Divide/1 -> Trigonometric Function/1
  Magnitude/1(|g|) -> Product/2, Divide/2
  Trigonometric Function2/1 -> Product/1
  Trigonometric Function/1 -> Gain/1
  y_acc/1 -> Magnitude/2(y_acc), Divide1/1
  z_acc/1 -> Magnitude/3(z_acc)
  Divide1/1 -> Trigonometric Function1/1
  Product/1 -> Divide1/2
  Trigonometric Function1/1 -> phi_acc/1  "phi_acc"
  x_acc/1 -> Magnitude/1(x_acc), Divide/1
  Gain/1 -> theta_acc/1, Trigonometric Function2/1  "theta_acc"

== system NLGC_1/On-board State Estimation/filterRawData()/Filter IC fixer ==
  FilterStart : Inport
  Normal Output : Inport  Port=2
  Constant : Constant
  IC : InitialCondition  Value=0
  Switch : Switch  Criteria=u2 ~= 0
  Out1 : Outport
  wires:
  Switch/1 -> Out1/1
  FilterStart/1 -> Switch/3
  IC/1 -> Switch/2
  Constant/1 -> IC/1
  Normal Output/1 -> Switch/1

== system NLGC_1/On-board State Estimation/filterRawData()/Filter IC fixer1 ==
  FilterStart : Inport
  Normal Output : Inport  Port=2
  Constant : Constant
  IC : InitialCondition  Value=0
  Switch : Switch  Criteria=u2 ~= 0
  Out1 : Outport
  wires:
  Switch/1 -> Out1/1
  FilterStart/1 -> Switch/3
  IC/1 -> Switch/2
  Constant/1 -> IC/1
  Normal Output/1 -> Switch/1

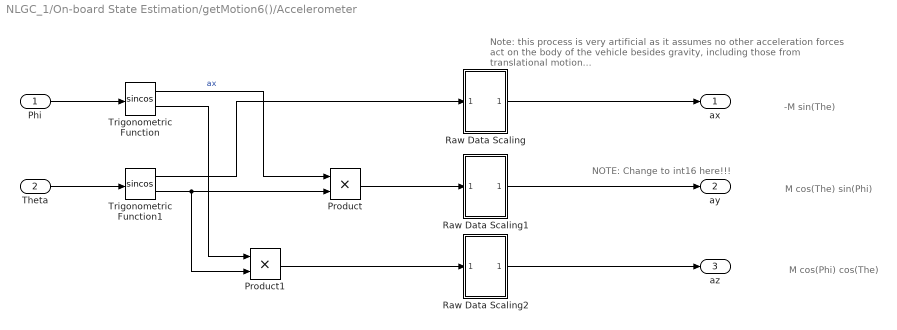
== system NLGC_1/On-board State Estimation/getMotion6()/Accelerometer ==
  note: NOTE: Change to int16 here!!!
  note: Note: this process is very artificial as it assumes no other acceleration
      | forces act on the body of the vehicle besides gravity, including those from
      | translational motion...
  note: -M sin(The)
  note: M cos(The) sin(Phi)
  note: M cos(Phi) cos(The)
  Phi : Inport
  Theta : Inport  Port=2
  Product : Product
  Product1 : Product
  Raw Data Scaling : Subsystem
  Raw Data Scaling1 : Subsystem
  Raw Data Scaling2 : Subsystem
  Trigonometric Function : Trigonometry  Operator=sincos  OutputSignalType=real
  Trigonometric Function1 : Trigonometry  Operator=sincos  OutputSignalType=real
  ax : Outport
  ay : Outport  Port=2
  az : Outport  Port=3
  wires:
  Phi/1 -> Trigonometric Function/1
  Theta/1 -> Trigonometric Function1/1
  Trigonometric Function/1 -> Product/1  "ax"
  Trigonometric Function1/2 -> Product1/2, Product/2
  Trigonometric Function/2 -> Product1/1
  Raw Data Scaling1/1(Out1) -> ay/1
  Raw Data Scaling2/1(Out1) -> az/1
  Product/1 -> Raw Data Scaling1/1(In1)
  Product1/1 -> Raw Data Scaling2/1(In1)
  Trigonometric Function1/1 -> Raw Data Scaling/1(In1)
  Raw Data Scaling/1(Out1) -> ax/1

== system NLGC_1/On-board State Estimation/getMotion6()/Gyro signals ==
  P : Inport
  Q : Inport  Port=2
  R : Inport  Port=3
  Gyro Raw Data Scaling : Subsystem
  Gyro Raw Data Scaling1 : Subsystem
  Gyro Raw Data Scaling2 : Subsystem
  gx : Outport
  gy : Outport  Port=2
  gz : Outport  Port=3
  wires:
  P/1 -> Gyro Raw Data Scaling/1(In1)
  Q/1 -> Gyro Raw Data Scaling1/1(In1)
  R/1 -> Gyro Raw Data Scaling2/1(In1)
  Gyro Raw Data Scaling/1(Out1) -> gx/1
  Gyro Raw Data Scaling1/1(Out1) -> gy/1
  Gyro Raw Data Scaling2/1(Out1) -> gz/1

== system NLGC_1/Quadcopter Dynamics/Motor Dynamics/Throttle To RPM Gain and Cutoff_1 ==
  note: minThr should be a quad.mat value
  note: This gain should be a quad.mat value
  note: This constant should be a quad.mat value
  note: Output equals linearly scaled RPM
      | for given throttle input if throttle input >=Throttle Cuttoff (minThr)
      | else output is zero.
  In5 : Inport
  Constant : Constant  Value=quadModel.b
  Gain : Gain  Gain=quadModel.cr
  Minimum Throttle Cutoff : simulink/Logic and Bit Operations/Compare To Constant  relop=>=  const=quadModel.minThr  OutDataTypeStr=uint8
  Product : Product
  Sum1 : Sum  Inputs=++|
  Out5 : Outport
  wires:
  Minimum Throttle Cutoff/1 -> Product/2
  Product/1 -> Out5/1
  In5/1 -> Gain/1, Minimum Throttle Cutoff/1
  Gain/1 -> Sum1/2
  Sum1/1 -> Product/1
  Constant/1 -> Sum1/1

== system NLGC_1/Quadcopter Dynamics/Motor Dynamics/Throttle To RPM Gain and Cutoff_2 ==
  note: minThr should be a quad.mat value
  note: This gain should be a quad.mat value
  note: This constant should be a quad.mat value
  note: Output equals linearly scaled RPM
      | for given throttle input if throttle input >=Throttle Cuttoff (minThr)
      | else output is zero.
  In5 : Inport
  Constant : Constant  Value=quadModel.b
  Gain : Gain  Gain=quadModel.cr
  Minimum Throttle Cutoff : simulink/Logic and Bit Operations/Compare To Constant  relop=>=  const=quadModel.minThr  OutDataTypeStr=uint8
  Product : Product
  Sum1 : Sum  Inputs=++|
  Out5 : Outport
  wires:
  Minimum Throttle Cutoff/1 -> Product/2
  Product/1 -> Out5/1
  In5/1 -> Gain/1, Minimum Throttle Cutoff/1
  Gain/1 -> Sum1/2
  Sum1/1 -> Product/1
  Constant/1 -> Sum1/1

== system NLGC_1/Quadcopter Dynamics/Motor Dynamics/Throttle To RPM Gain and Cutoff_3 ==
  note: minThr should be a quad.mat value
  note: This gain should be a quad.mat value
  note: This constant should be a quad.mat value
  note: Output equals linearly scaled RPM
      | for given throttle input if throttle input >=Throttle Cuttoff (minThr)
      | else output is zero.
  In5 : Inport
  Constant : Constant  Value=quadModel.b
  Gain : Gain  Gain=quadModel.cr
  Minimum Throttle Cutoff : simulink/Logic and Bit Operations/Compare To Constant  relop=>=  const=quadModel.minThr  OutDataTypeStr=uint8
  Product : Product
  Sum1 : Sum  Inputs=++|
  Out5 : Outport
  wires:
  Minimum Throttle Cutoff/1 -> Product/2
  Product/1 -> Out5/1
  In5/1 -> Gain/1, Minimum Throttle Cutoff/1
  Gain/1 -> Sum1/2
  Sum1/1 -> Product/1
  Constant/1 -> Sum1/1

== system NLGC_1/Quadcopter Dynamics/Motor Dynamics/Throttle To RPM Gain and Cutoff_4 ==
  note: minThr should be a quad.mat value
  note: This gain should be a quad.mat value
  note: This constant should be a quad.mat value
  note: Output equals linearly scaled RPM
      | for given throttle input if throttle input >=Throttle Cuttoff (minThr)
      | else output is zero.
  In5 : Inport
  Constant : Constant  Value=quadModel.b
  Gain : Gain  Gain=quadModel.cr
  Minimum Throttle Cutoff : simulink/Logic and Bit Operations/Compare To Constant  relop=>=  const=quadModel.minThr  OutDataTypeStr=uint8
  Product : Product
  Sum1 : Sum  Inputs=++|
  Out5 : Outport
  wires:
  Minimum Throttle Cutoff/1 -> Product/2
  Product/1 -> Out5/1
  In5/1 -> Gain/1, Minimum Throttle Cutoff/1
  Gain/1 -> Sum1/2
  Sum1/1 -> Product/1
  Constant/1 -> Sum1/1

== system NLGC_1/On-board State Estimation/State Estimation and Complimentary Mixing/Complimentary Filter/Filter IC fixer ==
  FilterStart : Inport
  Normal Output : Inport  Port=2
  Constant : Constant
  IC : InitialCondition  Value=0
  Switch : Switch  Criteria=u2 ~= 0  SampleTime=ControllerSampleTime
  Out1 : Outport
  wires:
  Switch/1 -> Out1/1
  FilterStart/1 -> Switch/3
  IC/1 -> Switch/2
  Constant/1 -> IC/1
  Normal Output/1 -> Switch/1

== system NLGC_1/On-board State Estimation/State Estimation and Complimentary Mixing/Complimentary Filter/Filter IC fixer1 ==
  FilterStart : Inport
  Normal Output : Inport  Port=2
  Constant : Constant
  IC : InitialCondition  Value=0
  Switch : Switch  Criteria=u2 ~= 0  SampleTime=ControllerSampleTime
  Out1 : Outport
  wires:
  Switch/1 -> Out1/1
  FilterStart/1 -> Switch/3
  IC/1 -> Switch/2
  Constant/1 -> IC/1
  Normal Output/1 -> Switch/1

== system NLGC_1/On-board State Estimation/State Estimation and Complimentary Mixing/Complimentary Filter/Filter IC fixer2 ==
  FilterStart : Inport
  Normal Output : Inport  Port=2
  Constant : Constant
  IC : InitialCondition  Value=0
  Switch : Switch  Criteria=u2 ~= 0  SampleTime=ControllerSampleTime
  Out1 : Outport
  wires:
  Switch/1 -> Out1/1
  FilterStart/1 -> Switch/3
  IC/1 -> Switch/2
  Constant/1 -> IC/1
  Normal Output/1 -> Switch/1

== system NLGC_1/On-board State Estimation/State Estimation and Complimentary Mixing/Subsystem/Filter IC fixer1 ==
  FilterStart : Inport
  Normal Output : Inport  Port=2
  Constant : Constant
  IC : InitialCondition  Value=0
  Switch : Switch  Criteria=u2 ~= 0  SampleTime=ControllerSampleTime
  Out1 : Outport
  wires:
  Switch/1 -> Out1/1
  FilterStart/1 -> Switch/3
  IC/1 -> Switch/2
  Constant/1 -> IC/1
  Normal Output/1 -> Switch/1

== system NLGC_1/On-board State Estimation/State Estimation and Complimentary Mixing/Subsystem/Filter IC fixer2 ==
  FilterStart : Inport
  Normal Output : Inport  Port=2
  Constant : Constant
  IC : InitialCondition  Value=0
  Switch : Switch  Criteria=u2 ~= 0  SampleTime=ControllerSampleTime
  Out1 : Outport
  wires:
  Switch/1 -> Out1/1
  FilterStart/1 -> Switch/3
  IC/1 -> Switch/2
  Constant/1 -> IC/1
  Normal Output/1 -> Switch/1

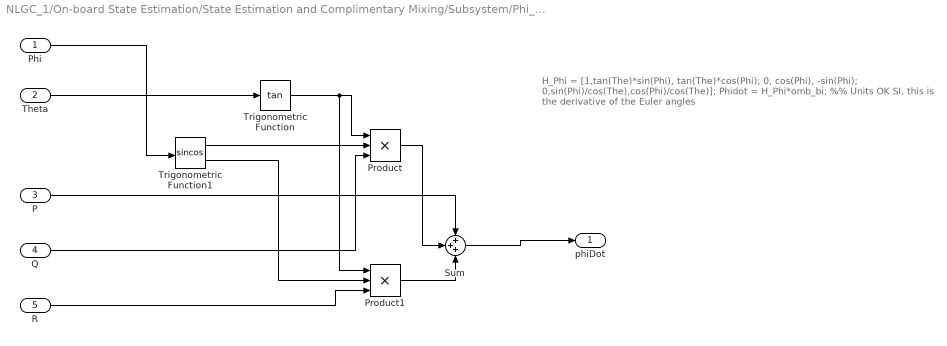
== system NLGC_1/On-board State Estimation/State Estimation and Complimentary Mixing/Subsystem/Phi_dot composer ==
  note: H_Phi = [1,tan(The)*sin(Phi), tan(The)*cos(Phi);
      |          0,         cos(Phi),         -sin(Phi);
      |          0,sin(Phi)/cos(The),cos(Phi)/cos(The)];
      | Phidot = H_Phi*omb_bi; %% Units OK SI, this is the derivative of the Euler angles
  Phi : Inport
  Theta : Inport  Port=2
  P : Inport  Port=3
  Q : Inport  Port=4
  R : Inport  Port=5
  Product : Product  Inputs=3
  Product1 : Product  Inputs=3
  Sum : Sum  Inputs=+++
  Trigonometric Function : Trigonometry  Operator=tan
  Trigonometric Function1 : Trigonometry  Operator=sincos
  phiDot : Outport
  wires:
  Sum/1 -> phiDot/1
  Trigonometric Function/1 -> Product1/1, Product/1
  Product1/1 -> Sum/3
  Q/1 -> Product/3
  Trigonometric Function1/1 -> Product/2
  Phi/1 -> Trigonometric Function1/1
  Theta/1 -> Trigonometric Function/1
  P/1 -> Sum/1
  R/1 -> Product1/3
  Product/1 -> Sum/2
  Trigonometric Function1/2 -> Product1/2

== system NLGC_1/On-board State Estimation/State Estimation and Complimentary Mixing/Subsystem/Phi_dot composer1 ==
  note: H_Phi = [1,tan(The)*sin(Phi), tan(The)*cos(Phi);
      |          0,         cos(Phi),         -sin(Phi);
      |          0,sin(Phi)/cos(The),cos(Phi)/cos(The)];
      | Phidot = H_Phi*omb_bi; %% Units OK SI
  Phi : Inport
  Theta : Inport  Port=2
  Q : Inport  Port=3
  R : Inport  Port=4
  Divide : Product  Inputs=**/
  Divide1 : Product  Inputs=**/
  Sum : Sum  Inputs=|++
  Trigonometric Function : Trigonometry  Operator=sincos
  Trigonometric Function1 : Trigonometry  Operator=cos
  psiDot : Outport
  wires:
  Sum/1 -> psiDot/1
  Phi/1 -> Trigonometric Function/1
  Trigonometric Function/1 -> Divide/2
  Theta/1 -> Trigonometric Function1/1
  Divide/1 -> Sum/1
  Trigonometric Function1/1 -> Divide/3, Divide1/3
  Q/1 -> Divide/1
  R/1 -> Divide1/2
  Divide1/1 -> Sum/2
  Trigonometric Function/2 -> Divide1/1

== system NLGC_1/On-board State Estimation/State Estimation and Complimentary Mixing/Subsystem/Theta_dot composer1 ==
  note: H_Phi = [1,tan(The)*sin(Phi), tan(The)*cos(Phi);
      |          0,         cos(Phi),         -sin(Phi);
      |          0,sin(Phi)/cos(The),cos(Phi)/cos(The)];
      | Phidot = H_Phi*omb_bi; %% Units OK SI
  Phi : Inport
  Q : Inport  Port=2
  R : Inport  Port=3
  Product : Product
  Product1 : Product
  Scope : Scope  NumInputPorts=2
  Sum : Sum  Inputs=|++
  Trigonometric Function2 : Trigonometry  Operator=sincos
  Unary Minus : UnaryMinus
  thetaDot : Outport
  wires:
  Sum/1 -> thetaDot/1
  Phi/1 -> Trigonometric Function2/1
  Q/1 -> Product/2
  Product/1 -> Sum/1
  Trigonometric Function2/1 -> Scope/2, Unary Minus/1
  Unary Minus/1 -> Scope/1, Product1/1
  R/1 -> Product1/2
  Product1/1 -> Sum/2
  Trigonometric Function2/2 -> Product/1

== system NLGC_1/On-board State Estimation/State Estimation and Complimentary Mixing/Subsystem1/Magnitude ==
  x_acc : Inport
  y_acc : Inport  Port=2
  z_acc : Inport  Port=3
  Demux1 : Demux  Outputs=3
  Math Function : Math  Operator=square  SaturateOnIntegerOverflow=on
  Mux : Mux  Inputs=3
  Sqrt : Sqrt  SaturateOnIntegerOverflow=on
  Sum : Sum  Inputs=+++
  |g| : Outport
  wires:
  Sqrt/1 -> |g|/1  "mag_acc"
  Sum/1 -> Sqrt/1
  Demux1/3 -> Sum/3
  Mux/1 -> Math Function/1
  Math Function/1 -> Demux1/1
  Demux1/1 -> Sum/1
  Demux1/2 -> Sum/2
  y_acc/1 -> Mux/2
  x_acc/1 -> Mux/1
  z_acc/1 -> Mux/3

== system NLGC_1/On-board State Estimation/getMotion6()/Accelerometer/Raw Data Scaling ==
  In1 : Inport
  Data Type Conversion : DataTypeConversion  OutDataTypeStr=int16  SaturateOnIntegerOverflow=on
  Gain1 : Gain  Gain=-16384  RndMeth=Round  SaturateOnIntegerOverflow=on
  Out1 : Outport
  wires:
  Gain1/1 -> Data Type Conversion/1
  In1/1 -> Gain1/1
  Data Type Conversion/1 -> Out1/1

== system NLGC_1/On-board State Estimation/getMotion6()/Accelerometer/Raw Data Scaling1 ==
  In1 : Inport
  Data Type Conversion : DataTypeConversion  OutDataTypeStr=int16
  Gain1 : Gain  Gain=16384  RndMeth=Round  SaturateOnIntegerOverflow=on
  Out1 : Outport
  wires:
  Gain1/1 -> Data Type Conversion/1
  In1/1 -> Gain1/1
  Data Type Conversion/1 -> Out1/1

== system NLGC_1/On-board State Estimation/getMotion6()/Accelerometer/Raw Data Scaling2 ==
  In1 : Inport
  Data Type Conversion : DataTypeConversion  OutDataTypeStr=int16
  Gain1 : Gain  Gain=16384  RndMeth=Round  SaturateOnIntegerOverflow=on
  Out1 : Outport
  wires:
  Gain1/1 -> Data Type Conversion/1
  In1/1 -> Gain1/1
  Data Type Conversion/1 -> Out1/1

== system NLGC_1/On-board State Estimation/getMotion6()/Gyro signals/Gyro Raw Data Scaling ==
  In1 : Inport
  Data Type Conversion : DataTypeConversion  OutDataTypeStr=int16  SaturateOnIntegerOverflow=on
  Gain1 : Gain  Gain=180*131.1/pi  RndMeth=Round  SaturateOnIntegerOverflow=on
  Out1 : Outport
  wires:
  Gain1/1 -> Data Type Conversion/1
  In1/1 -> Gain1/1
  Data Type Conversion/1 -> Out1/1

== system NLGC_1/On-board State Estimation/getMotion6()/Gyro signals/Gyro Raw Data Scaling1 ==
  In1 : Inport
  Data Type Conversion : DataTypeConversion  OutDataTypeStr=int16  SaturateOnIntegerOverflow=on
  Gain1 : Gain  Gain=180*131.1/pi  RndMeth=Round  SaturateOnIntegerOverflow=on
  Out1 : Outport
  wires:
  Gain1/1 -> Data Type Conversion/1
  In1/1 -> Gain1/1
  Data Type Conversion/1 -> Out1/1

== system NLGC_1/On-board State Estimation/getMotion6()/Gyro signals/Gyro Raw Data Scaling2 ==
  In1 : Inport
  Data Type Conversion : DataTypeConversion  OutDataTypeStr=int16  SaturateOnIntegerOverflow=on
  Gain1 : Gain  Gain=180*131.1/pi  RndMeth=Round  SaturateOnIntegerOverflow=on
  Out1 : Outport
  wires:
  Gain1/1 -> Data Type Conversion/1
  In1/1 -> Gain1/1
  Data Type Conversion/1 -> Out1/1
